simulink model "test1_v5"  (R2018a)
settings: Solver=VariableStepAuto  StartTime=0.0  StopTime=100  FixedStep=0.01  RelTol=1e-3  EnableMultiTasking=on
InitFcn:
  | run constants
values from neighbouring files (symbols this model uses):
  eul_0 = [tendeg tendeg tendeg]    [constants2.m]
  phi_noise = noise_att_on * noise_att_mag    [constants2.m]
  pm_0 = [0 0 0]    [constants2.m]
  Psi_noise = noise_att_on * noise_att_mag    [constants2.m]
  R = (RE + 700*1000)    (= 7078000)    [constants2.m]
  T_d = Td_on * [0.001 0.001 0.001]    [constants2.m]
  theta_noise = noise_att_on * noise_att_mag    [constants2.m]
undefined symbols (not defined in the file or in its folder): dt, dt_noise, n, phi_D, phi_I, phi_P, pqr_noise, Psi_D, Psi_I, Psi_P, theta_D, theta_I, theta_P
libraries: shared6dofsys x3, simulink x2, shared6dof x1, sharedTrackingLibrary x1
settings Model: PacingRate=1000  Creator=Matt  LastModifiedBy=matth
settings SolverCC: AutoInsertRateTranBlk=on
settings DataIOCC: SaveOutput=off  SaveTime=off
settings OptimizationCC: DefaultParameterBehavior=Inlined  InlineInvariantSignals=on  EnhancedBackFolding=on  PassReuseOutputArgsAs=Individual arguments  StateBitsets=on  DataBitsets=on  ZeroExternalMemoryAtStartup=off  ZeroInternalMemoryAtStartup=off  NoFixptDivByZeroProtection=on  LifeSpan=1  OptimizeBlockOrder=speed  DifferentSizesBufferReuse=on
settings DebuggingCC: ParameterTunabilityLossMsg=error
settings HardwareCC: ProdBitPerPointer=32  ProdBitPerSizeT=32  ProdBitPerPtrDiffT=32  ProdLargestAtomicFloat=None  ProdIntDivRoundTo=Floor  ProdWordSize=32  ProdHWDeviceType=Generic->Custom
settings SFSimCC: MATLABDynamicMemAlloc=off
settings RTWCC: SystemTargetFile=ert.tlc  TLCOptions=-p0  GenCodeOnly=on  TemplateMakefile=ert_default_tmf  GenerateReport=on  RTWVerbose=off  IncludeHyperlinkInReport=on  LaunchReport=on  GenerateTraceInfo=on  GenerateTraceReport=on  GenerateTraceReportSl=on  GenerateTraceReportSf=on  GenerateTraceReportEml=on
settings CodeAppCC: ForceParamTrailComments=on  IgnoreCustomStorageClasses=off  OperatorAnnotations=on  SimulinkDataObjDesc=on  SFDataObjDesc=on  CustomSymbolStrGlobalVar=rt$N$M  CustomSymbolStrType=$N$M  CustomSymbolStrFcn=$N$M$F  CustomSymbolStrMacro=$N$M  InsertBlockDesc=on
settings ERTTargetCC: TargetLangStandard=C99 (ISO)  CodeReplacementLibrary=ISO_C  GenerateSampleERTMain=on  IncludeMdlTerminateFcn=off  SuppressErrorStatus=on  SupportAbsoluteTime=off  SupportNonFinite=off  SupportComplex=off  PurelyIntegerCode=on  InlinedParameterPlacement=NonHierarchical  RootIOFormat=Structure reference  ERTCustomFileTemplate=example_file_process.tlc

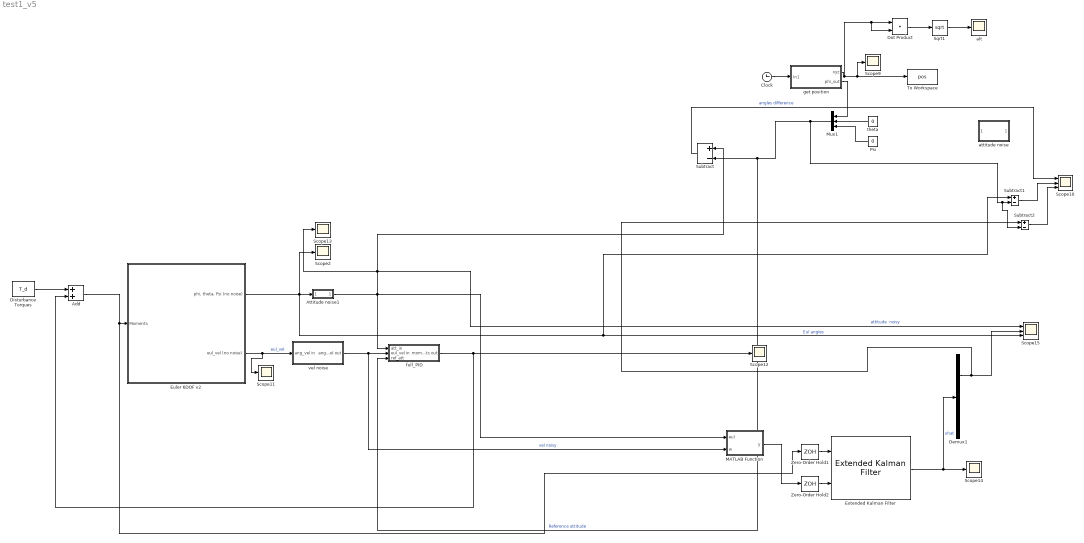
== system test1_v5 ==
  Add : Sum
  Attitude noise1 : Subsystem
  Clock : Clock
  Demux1 : Demux  Outputs=2
  Disturbance Torques : Constant  Value=T_d
  Dot Product : DotProduct  InputSameDT=on  OutDataTypeStr=Inherit: Inherit via internal rule
  Euler 6DOF v2 : Subsystem
  Extended Kalman Filter : sharedTrackingLibrary/Extended Kalman Filter  StateTransitionFcn=state_estimatation  HasStateTransitionJacobianFcn=off  HasAdditiveProcessNoise=Additive  ProcessNoise=state_covar  HasTimeVaryingProcessNoise=off  HasStateTransitionFcnExtraArgument=1  InitialState=state_init  InitialStateCovariance=init_covar  MeasurementFcn1=measure_func_fella  HasMeasurementJacobianFcn1=off  HasMeasurementEnablePort1=off  HasAdditiveMeasurementNoise1=Additive  MeasurementNoise1=measure_covar  HasTimeVaryingMeasurementNoise1=off  HasMeasurementFcnExtraArgument1=0  MeasurementFcn2=myMeasurementFcn  HasMeasurementJacobianFcn2=off  HasMeasurementEnablePort2=off  HasAdditiveMeasurementNoise2=Additive  MeasurementNoise2=1  HasTimeVaryingMeasurementNoise2=off  HasMeasurementFcnExtraArgument2=0  MeasurementFcn3=myMeasurementFcn  HasMeasurementJacobianFcn3=off  HasMeasurementEnablePort3=off  HasAdditiveMeasurementNoise3=Additive  MeasurementNoise3=1  HasTimeVaryingMeasurementNoise3=off  HasMeasurementFcnExtraArgument3=0  MeasurementFcn4=myMeasurementFcn  HasMeasurementJacobianFcn4=off  HasMeasurementEnablePort4=off  HasAdditiveMeasurementNoise4=Additive  MeasurementNoise4=1  HasTimeVaryingMeasurementNoise4=off  HasMeasurementFcnExtraArgument4=0  MeasurementFcn5=myMeasurementFcn  HasMeasurementJacobianFcn5=off  HasMeasurementEnablePort5=off  HasAdditiveMeasurementNoise5=Additive  MeasurementNoise5=1  HasTimeVaryingMeasurementNoise5=off  HasMeasurementFcnExtraArgument5=0  EnableMultirate=off  StateTransitionFcnSampleTime=1  MeasurementFcn1SampleTime=1  MeasurementFcn2SampleTime=1  MeasurementFcn3SampleTime=1  MeasurementFcn4SampleTime=1  MeasurementFcn5SampleTime=1  UseCurrentEstimator=off  OutputStateCovariance=off  DataType=double  SampleTime=dt  NumberOfMeasurements=1
      settings: SourceProductName=Control System Toolbox  SourceProductBaseCode=CT
  MATLAB Function : MATLAB Function  TreatAsAtomicUnit=on
  Mux1 : Mux  Inputs=3
  "Psi " : Constant  Value=0
  Scope10 : Scope  NumInputPorts=3
  Scope{2,9,11..14} (6 alike) : Scope
  Scope15 : Scope  NumInputPorts=3
  Sqrt1 : Sqrt  SaturateOnIntegerOverflow=on
  Subtract : Sum  Inputs=+-
  Subtract1 : Sum  Inputs=+-
  Subtract2 : Sum  Inputs=+-
  To Workspace : ToWorkspace  VariableName=pos  SaveFormat=Timeseries  SampleTime=-1
  Zero-Order Hold1 : ZeroOrderHold  SampleTime=dt
  Zero-Order Hold2 : ZeroOrderHold  SampleTime=dt
  alt : Scope
  attitude noise : Subsystem
  "full_PID " : Subsystem
  get position : Subsystem
  theta : Constant  Value=0
  "vel noise " : Subsystem
  wires:
  Euler 6DOF v2/1("phi, theta, Psi (no noise)") -> Subtract1/1, Scope15/3, Scope2/1, Attitude noise1/1(In1)  "Eul angles"
  Mux1/1 -> Subtract2/2, Subtract1/2, "full_PID "/3(ref_att), Subtract/2  "Reference attitude"
  "full_PID "/1(moments out) -> Add/2, Scope12/1
  Subtract/1 -> Scope10/1  "angles difference"
  Disturbance Torques/1 -> Add/1
  Add/1 -> Zero-Order Hold1/1, Euler 6DOF v2/1(Moments)
  Dot Product/1 -> Sqrt1/1
  Sqrt1/1 -> alt/1
  Clock/1 -> get position/1(In1)
  get position/1(xyz) -> Dot Product/2, Dot Product/1, To Workspace/1, Scope9/1
  Euler 6DOF v2/2(eul_vel (no noise)) -> Scope11/1, "vel noise "/1(ang_vel in)  "eul_vel"
  Attitude noise1/1(Out1) -> Subtract/1, Scope15/1, Scope13/1, MATLAB Function/1(eul), "full_PID "/1(att_in)  "attitude  noisy"
  "vel noise "/1(ang_vel out) -> MATLAB Function/2(w), "full_PID "/2(eul_vel in)  "vel noisy"
  get position/2(phi_out) -> Mux1/1
  "Psi "/1 -> Mux1/3
  theta/1 -> Mux1/2
  MATLAB Function/1(y) -> Zero-Order Hold2/1
  Zero-Order Hold1/1 -> Extended Kalman Filter/1
  Zero-Order Hold2/1 -> Extended Kalman Filter/2
  Extended Kalman Filter/1 -> Demux1/1, Scope14/1  "xhat"
  Demux1/1 -> Subtract2/1, Scope15/2
  Subtract1/1 -> Scope10/2
  Subtract2/1 -> Scope10/3

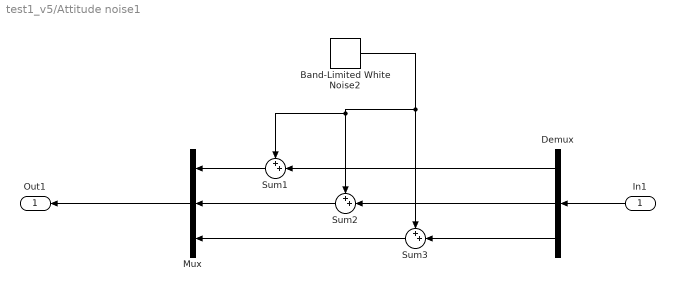
== system test1_v5/Attitude noise1 ==
  In1 : Inport
  Band-Limited White Noise2 : simulink/Sources/Band-Limited White Noise  Cov=3.0462e-6  Ts=dt_noise  seed=[23341]
  Demux : Demux  Outputs=3
  Mux : Mux  Inputs=3
  Sum1 : Sum  Inputs=++|
  Sum2 : Sum  Inputs=++|
  Sum3 : Sum  Inputs=++|
  Out1 : Outport
  wires:
  Demux/2 -> Sum2/2
  Demux/3 -> Sum3/2
  Sum2/1 -> Mux/2
  Sum3/1 -> Mux/3
  Sum1/1 -> Mux/1
  Band-Limited White Noise2/1 -> Sum1/1, Sum2/1, Sum3/1
  Demux/1 -> Sum1/2
  Mux/1 -> Out1/1
  In1/1 -> Demux/1

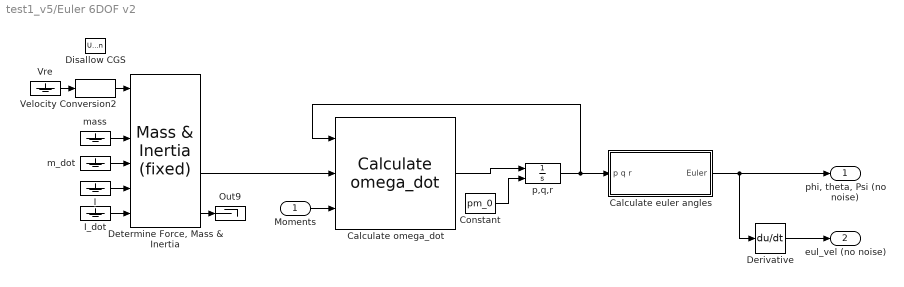
== system test1_v5/Euler 6DOF v2 ==
  Moments : Inport  Unit=N*m  PortDimensions=3
  Calculate euler angles : Subsystem
  Calculate omega_dot : shared6dofsys/Calculate omega_dot  aMode=aMode
      settings: SourceProductName=Aerospace Blockset  SourceProductBaseCode=AE
  Constant : Constant  Value=pm_0
  Derivative : Derivative
  "Determine Force, Mass & Inertia" : shared6dofsys/Mass & Inertia (fixed)  aMode=aMode
      settings: SourceProductName=Aerospace Blockset  SourceProductBaseCode=AE
  Disallow CGS : UnitConfiguration  UnitSystemsStr=English,SI,SI (extended)  AllowAllUnitSystems=off
  I : Ground
  I_dot : Ground
  Out9 : Terminator
  Velocity Conversion2 : shared6dof/6DOF (Euler Angles)/Velocity Conversion2
      settings: SourceProductName=Aerospace Blockset  SourceProductBaseCode=AE
  Vre : Ground
  m_dot : Ground
  mass : Ground
  "p,q,r " : Integrator  InitialConditionSource=external  InitialCondition=pm_0
  "phi, theta, Psi (no noise)" : Outport  Unit=rad
  eul_vel (no noise) : Outport  Port=2
  wires:
  Vre/1 -> Velocity Conversion2/1
  Calculate euler angles/1(Euler) -> Derivative/1, "phi, theta, Psi (no noise)"/1
  "p,q,r "/1 -> Calculate omega_dot/1, Calculate euler angles/1("p q r ")
  Moments/1 -> Calculate omega_dot/3
  "Determine Force, Mass & Inertia"/4 -> Out9/1
  mass/1 -> "Determine Force, Mass & Inertia"/3
  Calculate omega_dot/1 -> "p,q,r "/1
  I/1 -> "Determine Force, Mass & Inertia"/5
  "Determine Force, Mass & Inertia"/3 -> Calculate omega_dot/2
  Velocity Conversion2/1 -> "Determine Force, Mass & Inertia"/1
  I_dot/1 -> "Determine Force, Mass & Inertia"/6
  m_dot/1 -> "Determine Force, Mass & Inertia"/4
  Constant/1 -> "p,q,r "/2
  Derivative/1 -> eul_vel (no noise)/1

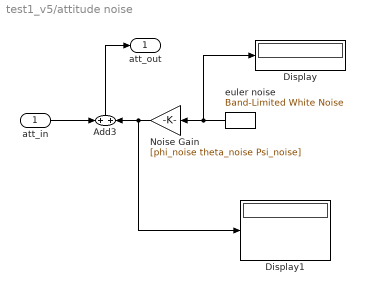
== system test1_v5/attitude noise ==
  att_in : Inport
  Add3 : Sum
  Display : Display
  Display1 : Display
  Noise Gain : Gain  Gain=[phi_noise theta_noise Psi_noise]
  euler noise : simulink/Sources/Band-Limited White Noise  Cov=0.1  Ts=0.1  seed=[23341]
  "att_out " : Outport
  wires:
  euler noise/1 -> Display/1, Noise Gain/1
  Noise Gain/1 -> Display1/1, Add3/2
  att_in/1 -> Add3/1
  Add3/1 -> "att_out "/1

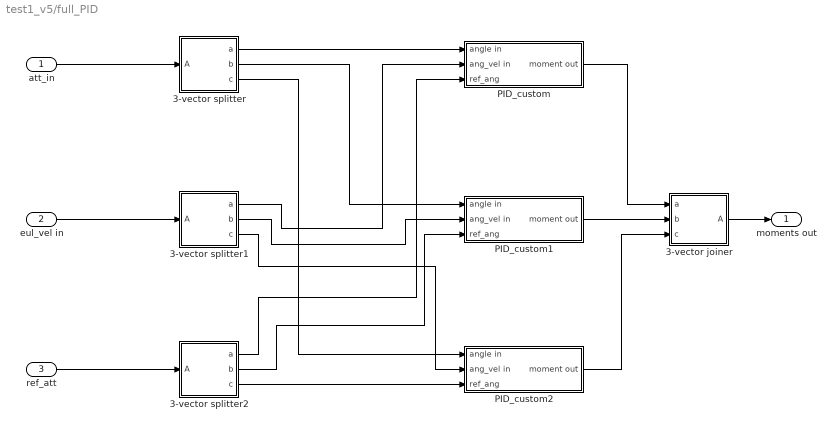
== system test1_v5/full_PID  ==
  att_in : Inport
  eul_vel in : Inport  Port=2
  ref_att : Inport  Port=3
  3-vector joiner : Subsystem
  3-vector splitter : Subsystem
  3-vector splitter1 : Subsystem
  3-vector splitter2 : Subsystem
  PID_custom : Subsystem
  PID_custom1 : Subsystem
  PID_custom2 : Subsystem
  moments out : Outport  InitialOutput=0
  wires:
  att_in/1 -> 3-vector splitter/1(A)
  eul_vel in/1 -> 3-vector splitter1/1(A)
  ref_att/1 -> 3-vector splitter2/1(A)
  3-vector splitter/1(a) -> PID_custom/1(angle in)
  3-vector splitter/2(b) -> PID_custom1/1(angle in)
  3-vector splitter/3(c) -> PID_custom2/1(angle in)
  3-vector splitter1/1(a) -> PID_custom/2(ang_vel in)
  3-vector splitter1/2(b) -> PID_custom1/2(ang_vel in)
  3-vector splitter1/3(c) -> PID_custom2/2(ang_vel in)
  3-vector splitter2/1(a) -> PID_custom/3("ref_ang ")
  3-vector splitter2/2(b) -> PID_custom1/3("ref_ang ")
  3-vector splitter2/3(c) -> PID_custom2/3("ref_ang ")
  PID_custom1/1("moment out ") -> 3-vector joiner/2(b)
  PID_custom/1("moment out ") -> 3-vector joiner/1(a)
  PID_custom2/1("moment out ") -> 3-vector joiner/3(c)
  3-vector joiner/1(A) -> moments out/1

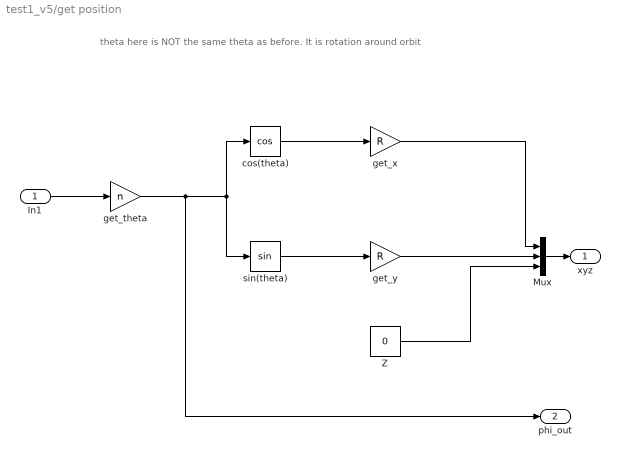
== system test1_v5/get position ==
  note: theta here is NOT the same theta as before. It is rotation around orbit
  In1 : Inport
  Mux : Mux  Inputs=3
  "Z " : Constant  Value=0
  cos(theta) : Trigonometry  Operator=cos
  get_theta : Gain  Gain=n
  "get_x " : Gain  Gain=R
  get_y : Gain  Gain=R
  sin(theta) : Trigonometry
  xyz : Outport
  phi_out : Outport  Port=2
  wires:
  In1/1 -> get_theta/1
  get_theta/1 -> phi_out/1, cos(theta)/1, sin(theta)/1
  cos(theta)/1 -> "get_x "/1
  sin(theta)/1 -> get_y/1
  "Z "/1 -> Mux/3
  get_y/1 -> Mux/2
  "get_x "/1 -> Mux/1
  Mux/1 -> xyz/1

== system test1_v5/vel noise  ==
  ang_vel in : Inport
  Add : Sum
  pqr_noise : Constant  Value=pqr_noise
  ang_vel out : Outport
  wires:
  ang_vel in/1 -> Add/2
  pqr_noise/1 -> Add/1
  Add/1 -> ang_vel out/1

== system test1_v5/Euler 6DOF v2/Calculate euler angles ==
  "p q r " : Inport
  phi theta psi : Integrator  InitialCondition=eul_0  WrapState=on
  phidot thetadot psidot : shared6dofsys/DCM & Euler Angles (Euler)/phidot thetadot psidot
      settings: SourceProductName=Aerospace Blockset  SourceProductBaseCode=AE
  Euler : Outport
  wires:
  "p q r "/1 -> phidot thetadot psidot/1
  phi theta psi/1 -> phidot thetadot psidot/2, Euler/1
  phidot thetadot psidot/1 -> phi theta psi/1

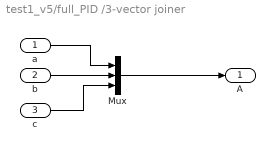
== system test1_v5/full_PID /3-vector joiner ==
  a : Inport
  b : Inport  Port=2
  c : Inport  Port=3
  Mux : Mux  Inputs=3
  A : Outport
  wires:
  c/1 -> Mux/3
  a/1 -> Mux/1
  b/1 -> Mux/2
  Mux/1 -> A/1

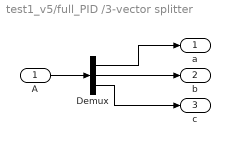
== system test1_v5/full_PID /3-vector splitter ==
  A : Inport
  Demux : Demux  Outputs=3
  a : Outport
  b : Outport  Port=2
  c : Outport  Port=3
  wires:
  Demux/3 -> c/1
  Demux/2 -> b/1
  Demux/1 -> a/1
  A/1 -> Demux/1

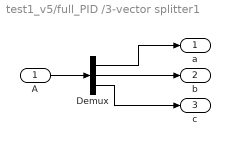
== system test1_v5/full_PID /3-vector splitter1 ==
  A : Inport
  Demux : Demux  Outputs=3
  a : Outport
  b : Outport  Port=2
  c : Outport  Port=3
  wires:
  Demux/3 -> c/1
  Demux/2 -> b/1
  Demux/1 -> a/1
  A/1 -> Demux/1

== system test1_v5/full_PID /3-vector splitter2 ==
  A : Inport
  Demux : Demux  Outputs=3
  a : Outport
  b : Outport  Port=2
  c : Outport  Port=3
  wires:
  Demux/3 -> c/1
  Demux/2 -> b/1
  Demux/1 -> a/1
  A/1 -> Demux/1

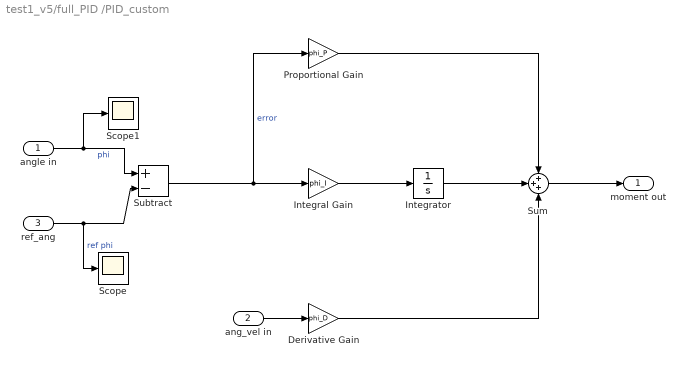
== system test1_v5/full_PID /PID_custom ==
  angle in : Inport
  ang_vel in : Inport  Port=2
  "ref_ang " : Inport  Port=3
  Derivative Gain : Gain  Gain=phi_D
  Integral Gain : Gain  Gain=phi_I
  Integrator : Integrator
  Proportional Gain : Gain  Gain=phi_P
  Scope : Scope
  Scope1 : Scope
  Subtract : Sum  Inputs=+-
  Sum : Sum  Inputs=+++
  "moment out " : Outport
  wires:
  angle in/1 -> Scope1/1, Subtract/1  "phi"
  "ref_ang "/1 -> Scope/1, Subtract/2  "ref phi"
  Subtract/1 -> Integral Gain/1, Proportional Gain/1  "error"
  Integral Gain/1 -> Integrator/1
  Proportional Gain/1 -> Sum/1
  Integrator/1 -> Sum/2
  ang_vel in/1 -> Derivative Gain/1
  Derivative Gain/1 -> Sum/3
  Sum/1 -> "moment out "/1

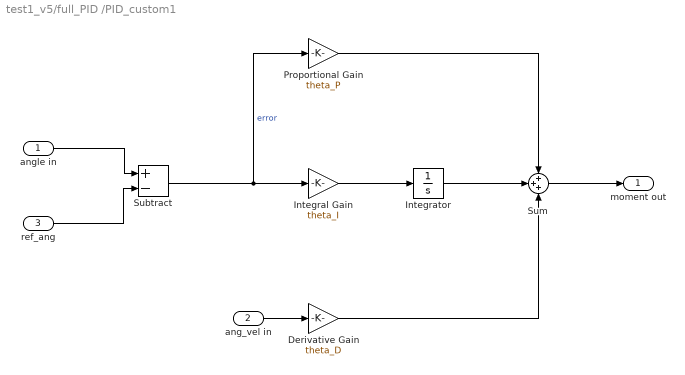
== system test1_v5/full_PID /PID_custom1 ==
  angle in : Inport
  ang_vel in : Inport  Port=2
  "ref_ang " : Inport  Port=3
  Derivative Gain : Gain  Gain=theta_D
  Integral Gain : Gain  Gain=theta_I
  Integrator : Integrator
  Proportional Gain : Gain  Gain=theta_P
  Subtract : Sum  Inputs=+-
  Sum : Sum  Inputs=+++
  "moment out " : Outport
  wires:
  angle in/1 -> Subtract/1
  "ref_ang "/1 -> Subtract/2
  Subtract/1 -> Integral Gain/1, Proportional Gain/1  "error"
  Integral Gain/1 -> Integrator/1
  Proportional Gain/1 -> Sum/1
  Integrator/1 -> Sum/2
  ang_vel in/1 -> Derivative Gain/1
  Derivative Gain/1 -> Sum/3
  Sum/1 -> "moment out "/1

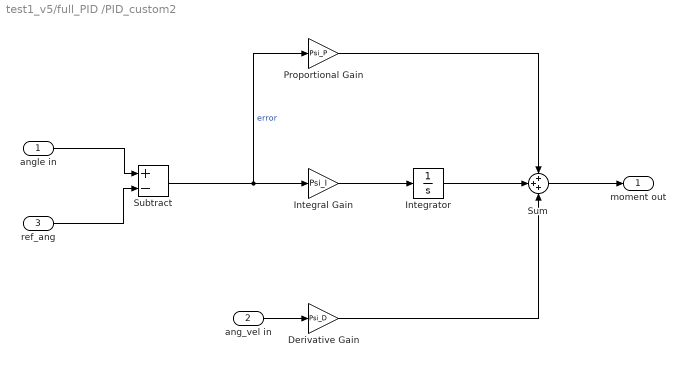
== system test1_v5/full_PID /PID_custom2 ==
  angle in : Inport
  ang_vel in : Inport  Port=2
  "ref_ang " : Inport  Port=3
  Derivative Gain : Gain  Gain=Psi_D
  Integral Gain : Gain  Gain=Psi_I
  Integrator : Integrator
  Proportional Gain : Gain  Gain=Psi_P
  Subtract : Sum  Inputs=+-
  Sum : Sum  Inputs=+++
  "moment out " : Outport
  wires:
  angle in/1 -> Subtract/1
  "ref_ang "/1 -> Subtract/2
  Subtract/1 -> Integral Gain/1, Proportional Gain/1  "error"
  Integral Gain/1 -> Integrator/1
  Proportional Gain/1 -> Sum/1
  Integrator/1 -> Sum/2
  ang_vel in/1 -> Derivative Gain/1
  Derivative Gain/1 -> Sum/3
  Sum/1 -> "moment out "/1

== matlab function test1_v5/MATLAB Function ==
  data: eul input; y output; w input
function y = get_state(eul, w)

y = [eul(1) eul(2) eul(3) w(1) w(2) w(3)];
end
